simulink model "callfunction"  (R2014a)
settings: Solver=ode45  StartTime=0.0  StopTime=10.0  RelTol=1e-3
settings Model: Creator=gxnuhuang  LastModifiedBy=gxnuhuang

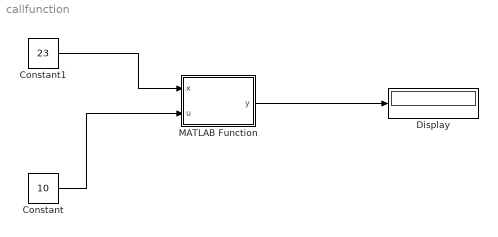
== system callfunction ==
  Constant : Constant  Value=10
  Constant1 : Constant  Value=23
  Display : Display
  MATLAB Function : MATLAB Function  TreatAsAtomicUnit=on
  wires:
  Constant1/1 -> MATLAB Function/1(x)
  Constant/1 -> MATLAB Function/2(u)
  MATLAB Function/1(y) -> Display/1

== matlab function callfunction/MATLAB Function ==
  data: x input; u input; y output
function y = testfuction(x,u)
%#codegen

y = u*x+1;
%fprintf('hzq:x=%d,u=%d,y=%d\n',x,u,y);
end
